simulink model "tocdo2"  (R2018b)
settings: Solver=FixedStepAuto  StartTime=0.0  StopTime=3  FixedStep=0.0003  RelTol=1e-3
undefined symbols (not defined in the file): J, KE, Ki, Kiv, Kp, Kpv, KT, La, Ra, Td, Tf, Tsp
settings Model: Creator=User  LastModifiedBy=User

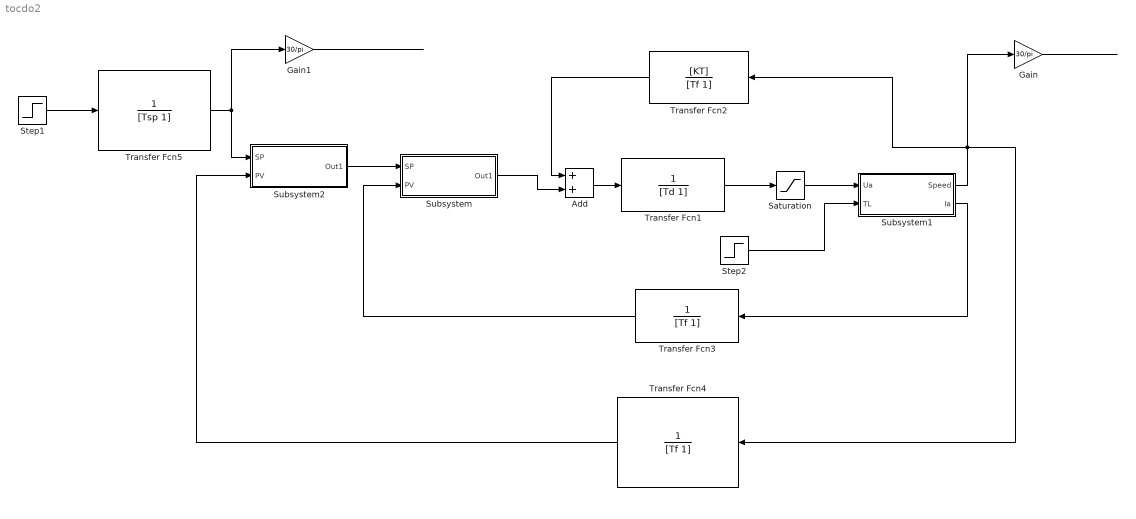
== system tocdo2 ==
  Add : Sum
  Gain : Gain  Gain=30/pi
  Gain1 : Gain  Gain=30/pi
  Saturation : Saturate  UpperLimit=350  LowerLimit=-350
  Step1 : Step  Time=0  After=2500*pi/30  SampleTime=0
  Step2 : Step  After=70  SampleTime=0
  Subsystem : Subsystem
  Subsystem1 : Subsystem
  Subsystem2 : Subsystem
  Transfer Fcn1 : TransferFcn  Denominator=[Td 1]
  Transfer Fcn2 : TransferFcn  Numerator=[KT]  Denominator=[Tf 1]
  Transfer Fcn3 : TransferFcn  Denominator=[Tf 1]
  Transfer Fcn4 : TransferFcn  Denominator=[Tf 1]
  Transfer Fcn5 : TransferFcn  Denominator=[Tsp 1]
  wires:
  Transfer Fcn3/1 -> Subsystem/2(PV)
  Subsystem1/2(Ia) -> Transfer Fcn3/1
  Step2/1 -> Subsystem1/2(TL)
  Add/1 -> Transfer Fcn1/1
  Subsystem/1(Out1) -> Add/2
  Transfer Fcn2/1 -> Add/1
  Subsystem1/1(Speed) -> Gain/1, Transfer Fcn2/1, Transfer Fcn4/1
  Transfer Fcn4/1 -> Subsystem2/2(PV)
  Subsystem2/1(Out1) -> Subsystem/1(SP)
  Transfer Fcn5/1 -> Subsystem2/1(SP), Gain1/1
  Step1/1 -> Transfer Fcn5/1
  Transfer Fcn1/1 -> Saturation/1
  Gain/1 -> ?
  Gain1/1 -> ?
  Saturation/1 -> Subsystem1/1(Ua)

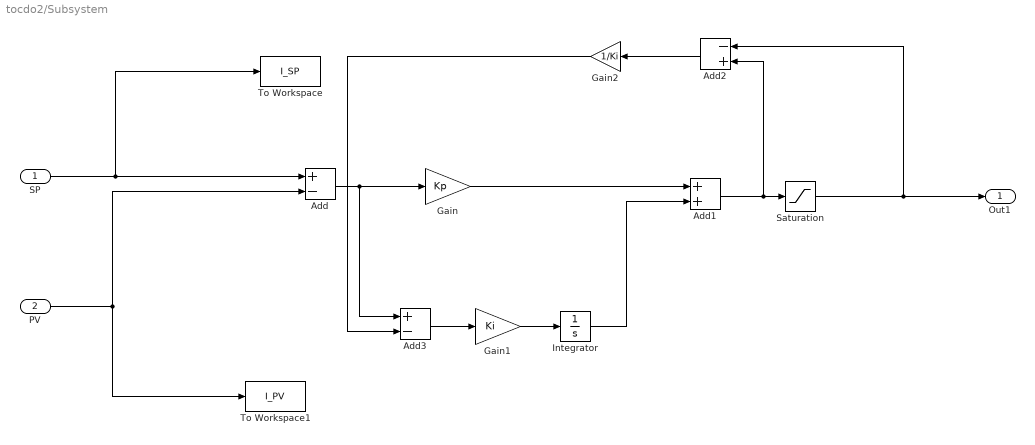
== system tocdo2/Subsystem ==
  SP : Inport
  PV : Inport  Port=2
  Add : Sum  Inputs=+-
  Add1 : Sum
  Add2 : Sum  Inputs=-+
  Add3 : Sum  Inputs=+-
  Gain : Gain  Gain=Kp
  Gain1 : Gain  Gain=Ki
  Gain2 : Gain  Gain=1/Ki
  Integrator : Integrator
  Saturation : Saturate  UpperLimit=200  LowerLimit=-200
  To Workspace : ToWorkspace  VariableName=I_SP  SaveFormat=Timeseries  SampleTime=-1
  To Workspace1 : ToWorkspace  VariableName=I_PV  SaveFormat=Timeseries  SampleTime=-1
  Out1 : Outport
  wires:
  SP/1 -> To Workspace/1, Add/1
  PV/1 -> Add/2, To Workspace1/1
  Add/1 -> Add3/1, Gain/1
  Gain1/1 -> Integrator/1
  Gain/1 -> Add1/1
  Integrator/1 -> Add1/2
  Add1/1 -> Add2/2, Saturation/1
  Saturation/1 -> Add2/1, Out1/1
  Add2/1 -> Gain2/1
  Gain2/1 -> Add3/2
  Add3/1 -> Gain1/1

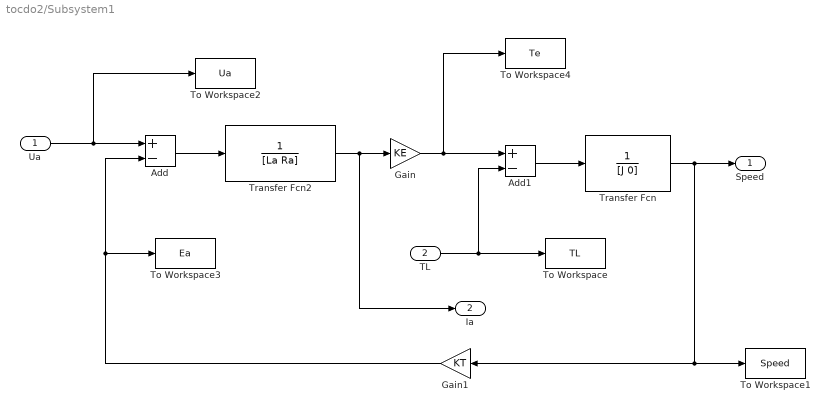
== system tocdo2/Subsystem1 ==
  Ua : Inport
  TL : Inport  Port=2
  Add : Sum  Inputs=+-
  Add1 : Sum  Inputs=+-
  Gain : Gain  Gain=KE
  Gain1 : Gain  Gain=KT
  To Workspace : ToWorkspace  VariableName=TL  SaveFormat=Timeseries  SampleTime=-1
  To Workspace1 : ToWorkspace  VariableName=Speed  SaveFormat=Timeseries  SampleTime=-1
  To Workspace2 : ToWorkspace  VariableName=Ua  SaveFormat=Timeseries  SampleTime=-1
  To Workspace3 : ToWorkspace  VariableName=Ea  SaveFormat=Timeseries  SampleTime=-1
  To Workspace4 : ToWorkspace  VariableName=Te  SaveFormat=Timeseries  SampleTime=-1
  Transfer Fcn : TransferFcn  Denominator=[J 0]
  Transfer Fcn2 : TransferFcn  Denominator=[La Ra]
  Speed : Outport
  Ia : Outport  Port=2
  wires:
  Add/1 -> Transfer Fcn2/1
  Transfer Fcn2/1 -> Ia/1, Gain/1
  Gain/1 -> To Workspace4/1, Add1/1
  Add1/1 -> Transfer Fcn/1
  Transfer Fcn/1 -> Gain1/1, To Workspace1/1, Speed/1
  TL/1 -> Add1/2, To Workspace/1
  Gain1/1 -> To Workspace3/1, Add/2
  Ua/1 -> To Workspace2/1, Add/1

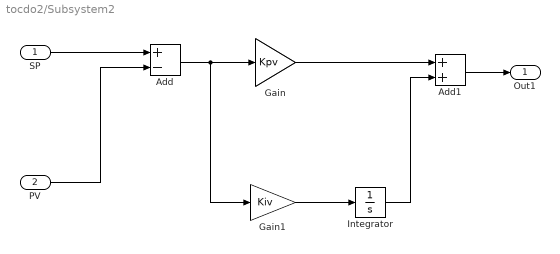
== system tocdo2/Subsystem2 ==
  SP : Inport
  PV : Inport  Port=2
  Add : Sum  Inputs=+-
  Add1 : Sum
  Gain : Gain  Gain=Kpv
  Gain1 : Gain  Gain=Kiv
  Integrator : Integrator
  Out1 : Outport
  wires:
  Add1/1 -> Out1/1
  Integrator/1 -> Add1/2
  Gain/1 -> Add1/1
  Gain1/1 -> Integrator/1
  Add/1 -> Gain/1, Gain1/1
  PV/1 -> Add/2
  SP/1 -> Add/1
